simulink model "Tugas_no_3"  (R2022b)
settings: Solver=VariableStepAuto  StartTime=0.0  StopTime=10.0  RelTol=1e-3
settings Model: Creator=hp  LastModifiedBy=hp

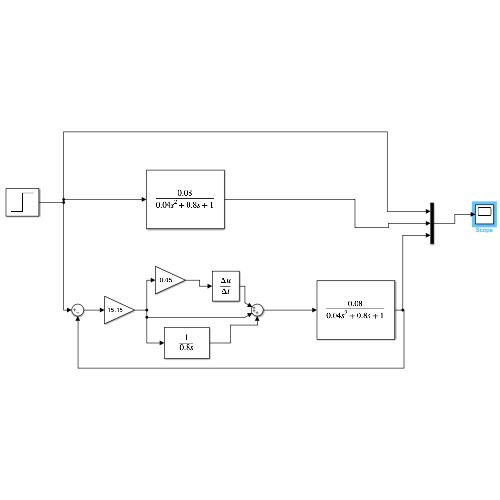
[thumbnail: Simulink's stored preview of the top-level diagram]
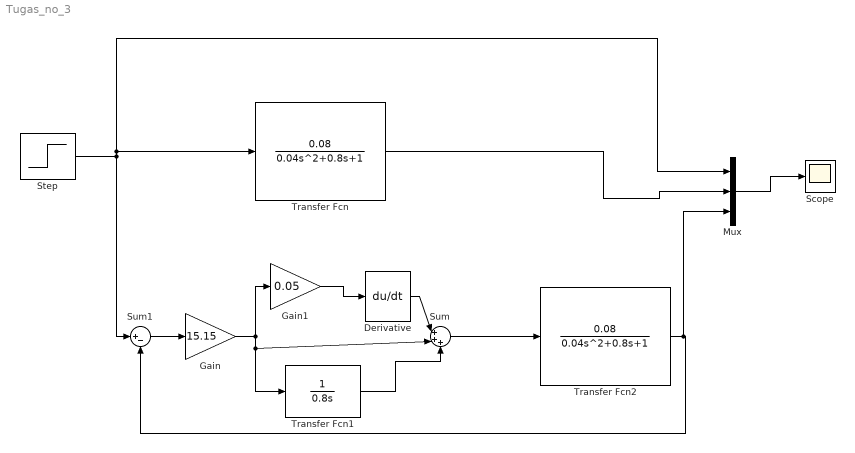
== system Tugas_no_3 ==
  Derivative : Derivative
  Gain : Gain  Gain=15.15
  Gain1 : Gain  Gain=0.05
  Mux : Mux  Inputs=3
  Scope : Scope
  Step : Step  SampleTime=0
  Sum : Sum  Inputs=|+++
  Sum1 : Sum  Inputs=|+-
  Transfer Fcn : TransferFcn  Numerator=[0.08]  Denominator=[0.04 0.8 1]
  Transfer Fcn1 : TransferFcn  Numerator=[1 ]  Denominator=[0.8 0]
  Transfer Fcn2 : TransferFcn  Numerator=[0.08]  Denominator=[0.04 0.8 1]
  wires:
  Mux/1 -> Scope/1
  Gain/1 -> Sum/2, Transfer Fcn1/1, Gain1/1
  Sum1/1 -> Gain/1
  Step/1 -> Mux/1, Transfer Fcn/1, Sum1/1
  Sum/1 -> Transfer Fcn2/1
  Transfer Fcn2/1 -> Sum1/2, Mux/3
  Transfer Fcn/1 -> Mux/2
  Transfer Fcn1/1 -> Sum/3
  Gain1/1 -> Derivative/1
  Derivative/1 -> Sum/1
